simulink model "PMSMSim"  (R2016a)
settings: Solver=ode4  StartTime=0.0  StopTime=2  FixedStep=0.0001  RelTol=1e-3
settings Model: Creator=B210b  LastModifiedBy=B210b

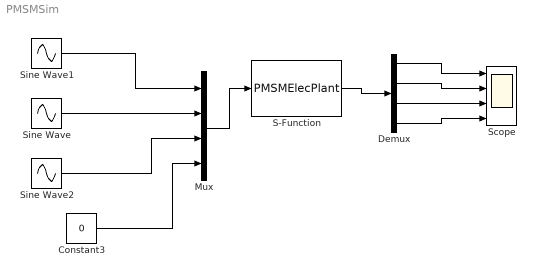
== system PMSMSim ==
  Constant3 : Constant  Value=0
  Demux : Demux
  Mux : Mux
  S-Function : S-Function  FunctionName=PMSMElecPlant  SFunctionDeploymentMode=off  EnableBusSupport=off
  Scope : Scope  NumInputPorts=4
  Sine Wave : Sin  Amplitude=220*sqrt(2)  Frequency=100*pi  SampleTime=0
  Sine Wave1 : Sin  Amplitude=220*sqrt(2)  Frequency=100*pi  Phase=-2/3*pi  SampleTime=0
  Sine Wave2 : Sin  Amplitude=220*sqrt(2)  Frequency=100*pi  Phase=2/3*pi  SampleTime=0
  wires:
  Mux/1 -> S-Function/1
  Sine Wave1/1 -> Mux/1
  Sine Wave/1 -> Mux/2
  Constant3/1 -> Mux/4
  S-Function/1 -> Demux/1
  Demux/1 -> Scope/1
  Demux/2 -> Scope/2
  Demux/3 -> Scope/3
  Demux/4 -> Scope/4
  Sine Wave2/1 -> Mux/3
